simulink model "aircraft_control_model_v2"  (R2020b)
settings: Solver=ode1be  StartTime=0.0  StopTime=t  RelTol=1e-3
values from neighbouring files (symbols this model uses):
  A_ce_CG_14 = A_ce_CG_14(2:3,2:3)    [aircraft_control_model_initialisation_v2.m]
  A_ce_CG_24 = A_ce_CG_24(2:3,2:3)    [aircraft_control_model_initialisation_v2.m]
  A_ce_CG_34 = A_ce_CG_34(2:3,2:3)    [aircraft_control_model_initialisation_v2.m]
  A_sc_CG_10 = A_sc_CG_10(2:3,2:3)    [aircraft_control_model_initialisation_v2.m]
  A_sc_CG_22 = A_sc_CG_22(2:3,2:3)    [aircraft_control_model_initialisation_v2.m]
  A_sc_CG_29 = A_sc_CG_29(2:3,2:3)    [aircraft_control_model_initialisation_v2.m]
  A_sc_CG_36 = A_sc_CG_36(2:3,2:3)    [aircraft_control_model_initialisation_v2.m]
  A_sc_CG_55 = A_sc_CG_55(2:3,2:3)    [aircraft_control_model_initialisation_v2.m]
  actuator_rate = 115*pi/180    (= 2.00712863979)    [aircraft_control_model_initialisation_v2.m]
  ail_sat = 30*pi/180    (= 0.523598775598)    [aircraft_control_model_initialisation_v2.m]
  alpha0 = base_scout_aircraft_constants(16)    [aircraft_control_model_initialisation_v2.m]
  alpha0_ce = base_cessna_aircraft_constants(16)    [aircraft_control_model_initialisation_v2.m]
  alpha0tot_ce_CG_14 = consts_ce_CG_14(17)    [aircraft_control_model_initialisation_v2.m]
  alpha0tot_ce_CG_24 = consts_ce_CG_24(17)    [aircraft_control_model_initialisation_v2.m]
  alpha0tot_ce_CG_34 = consts_ce_CG_34(17)    [aircraft_control_model_initialisation_v2.m]
  alpha0tot_sc_CG_10 = consts_sc_CG_10(17)    [aircraft_control_model_initialisation_v2.m]
  alpha0tot_sc_CG_22 = consts_sc_CG_22(17)    [aircraft_control_model_initialisation_v2.m]
  alpha0tot_sc_CG_29 = consts_sc_CG_29(17)    [aircraft_control_model_initialisation_v2.m]
  alpha0tot_sc_CG_36 = consts_sc_CG_36(17)    [aircraft_control_model_initialisation_v2.m]
  alpha0tot_sc_CG_55 = consts_sc_CG_55(17)    [aircraft_control_model_initialisation_v2.m]
  alpha_ts = base_scout_aircraft_constants(19)    [aircraft_control_model_initialisation_v2.m]
  alpha_ts_ce = base_cessna_aircraft_constants(19)    [aircraft_control_model_initialisation_v2.m]
  alpha_ws = base_scout_aircraft_constants(18)    [aircraft_control_model_initialisation_v2.m]
  alpha_ws_ce = base_cessna_aircraft_constants(18)    [aircraft_control_model_initialisation_v2.m]
  AR_w = base_scout_aircraft_constants(8)    [aircraft_control_model_initialisation_v2.m]
  AR_w_ce = base_cessna_aircraft_constants(8)    [aircraft_control_model_initialisation_v2.m]
  b1 = base_scout_aircraft_constants(23)    [aircraft_control_model_initialisation_v2.m]
  b1_ce = base_cessna_aircraft_constants(23)    [aircraft_control_model_initialisation_v2.m]
  b2 = base_scout_aircraft_constants(24)    [aircraft_control_model_initialisation_v2.m]
  b2_ce = base_cessna_aircraft_constants(24)    [aircraft_control_model_initialisation_v2.m]
  b3 = base_scout_aircraft_constants(25)    [aircraft_control_model_initialisation_v2.m]
  b3_ce = base_cessna_aircraft_constants(25)    [aircraft_control_model_initialisation_v2.m]
  B_ce_CG_14 = B_ce_CG_14(2:3,1:1)    [aircraft_control_model_initialisation_v2.m]
  B_ce_CG_24 = B_ce_CG_24(2:3,1:1)    [aircraft_control_model_initialisation_v2.m]
  B_ce_CG_34 = B_ce_CG_34(2:3,1:1)    [aircraft_control_model_initialisation_v2.m]
  B_sc = B_sc(:,1)    [aircraft_control_model_initialisation_v2.m]
  B_sc_CG_10 = B_sc_CG_10(2:3,1:1)    [aircraft_control_model_initialisation_v2.m]
  B_sc_CG_22 = B_sc_CG_22(2:3,1:1)    [aircraft_control_model_initialisation_v2.m]
  B_sc_CG_29 = B_sc_CG_29(2:3,1:1)    [aircraft_control_model_initialisation_v2.m]
  B_sc_CG_36 = B_sc_CG_36(2:3,1:1)    [aircraft_control_model_initialisation_v2.m]
  B_sc_CG_55 = B_sc_CG_55(2:3,1:1)    [aircraft_control_model_initialisation_v2.m]
  beta_ce_CG_14 = consts_ce_CG_14(21)    [aircraft_control_model_initialisation_v2.m]
  beta_ce_CG_24 = consts_ce_CG_24(21)    [aircraft_control_model_initialisation_v2.m]
  beta_ce_CG_34 = consts_ce_CG_34(21)    [aircraft_control_model_initialisation_v2.m]
  beta_sc_CG_10 = consts_sc_CG_10(21)    [aircraft_control_model_initialisation_v2.m]
  beta_sc_CG_22 = consts_sc_CG_22(21)    [aircraft_control_model_initialisation_v2.m]
  beta_sc_CG_29 = consts_sc_CG_29(21)    [aircraft_control_model_initialisation_v2.m]
  beta_sc_CG_36 = consts_sc_CG_36(21)    [aircraft_control_model_initialisation_v2.m]
  beta_sc_CG_55 = consts_sc_CG_55(21)    [aircraft_control_model_initialisation_v2.m]
  c_e = base_scout_aircraft_constants(10)    [aircraft_control_model_initialisation_v2.m]
  c_e_ce = base_cessna_aircraft_constants(10)    [aircraft_control_model_initialisation_v2.m]
  Cm0 = base_scout_aircraft_constants(11)    [aircraft_control_model_initialisation_v2.m]
  control_surface_feedback = 10    [aircraft_control_model_initialisation_v2.m]
  dCL_w_dalpha = base_scout_aircraft_constants(14)    [aircraft_control_model_initialisation_v2.m]
  dCL_w_dalpha_ce = base_cessna_aircraft_constants(14)    [aircraft_control_model_initialisation_v2.m]
  dCLtot_dalpha = base_scout_aircraft_constants(15)    [aircraft_control_model_initialisation_v2.m]
  dCLtot_dalpha_ce = base_cessna_aircraft_constants(15)    [aircraft_control_model_initialisation_v2.m]
  dt = 1/100    (= 0.01)    [aircraft_control_model_initialisation_v2.m]
  elev_amplitude = 15*pi/180    (= 0.261799387799)    [aircraft_control_model_initialisation_v2.m]
  elev_cutoff = 35*pi/180    (= 0.610865238198)    [aircraft_control_model_initialisation_v2.m]
  elev_period = 1    [aircraft_control_model_initialisation_v2.m]
  elev_period_start = 5    [aircraft_control_model_initialisation_v2.m]
  elev_sat = 28*pi/180    (= 0.488692190558)    [aircraft_control_model_initialisation_v2.m]
  eta_ce_CG_14 = consts_ce_CG_14(22)    [aircraft_control_model_initialisation_v2.m]
  eta_ce_CG_24 = consts_ce_CG_24(22)    [aircraft_control_model_initialisation_v2.m]
  eta_ce_CG_34 = consts_ce_CG_34(22)    [aircraft_control_model_initialisation_v2.m]
  eta_sc_CG_10 = consts_sc_CG_10(22)    [aircraft_control_model_initialisation_v2.m]
  eta_sc_CG_22 = consts_sc_CG_22(22)    [aircraft_control_model_initialisation_v2.m]
  eta_sc_CG_29 = consts_sc_CG_29(22)    [aircraft_control_model_initialisation_v2.m]
  eta_sc_CG_36 = consts_sc_CG_36(22)    [aircraft_control_model_initialisation_v2.m]
  eta_sc_CG_55 = consts_sc_CG_55(22)    [aircraft_control_model_initialisation_v2.m]
  g = base_scout_aircraft_constants(3)    [aircraft_control_model_initialisation_v2.m]
  G = base_scout_aircraft_constants(26)    [aircraft_control_model_initialisation_v2.m]
  g_ce = base_cessna_aircraft_constants(3)    [aircraft_control_model_initialisation_v2.m]
  G_ce = base_cessna_aircraft_constants(26)    [aircraft_control_model_initialisation_v2.m]
  h0 = base_scout_aircraft_constants(13)    [aircraft_control_model_initialisation_v2.m]
  h_cg = base_scout_aircraft_constants(12)    [aircraft_control_model_initialisation_v2.m]
  K = base_scout_aircraft_constants(7)    [aircraft_control_model_initialisation_v2.m]
  l_m = base_scout_aircraft_constants(27)    [aircraft_control_model_initialisation_v2.m]
  l_m_ce = base_cessna_aircraft_constants(27)    [aircraft_control_model_initialisation_v2.m]
  m = base_scout_aircraft_constants(2)    [aircraft_control_model_initialisation_v2.m]
  m_ce = base_cessna_aircraft_constants(2)    [aircraft_control_model_initialisation_v2.m]
  modM = base_scout_aircraft_constants(30)    [aircraft_control_model_initialisation_v2.m]
  modM_ce = base_cessna_aircraft_constants(30)    [aircraft_control_model_initialisation_v2.m]
  n = base_scout_aircraft_constants(1)    [aircraft_control_model_initialisation_v2.m]    (also in xplane_data_decoder.m = data_input(6,2))
  ppgain_actuator_D = 1.076123507883140e+02    (= 107.612350788)    [aircraft_control_model_initialisation_v2.m]
  ppgain_actuator_P = 20.729870007825970    (= 20.7298700078)    [aircraft_control_model_initialisation_v2.m]
  ppgain_D = 0.637114873357555    (= 0.637114873358)    [aircraft_control_model_initialisation_v2.m]
  ppgain_P = -86.717674561182620    (= -86.7176745612)    [aircraft_control_model_initialisation_v2.m]
  r = base_scout_aircraft_constants(29)    [aircraft_control_model_initialisation_v2.m]
  r_ce = base_cessna_aircraft_constants(29)    [aircraft_control_model_initialisation_v2.m]
  rho = base_scout_aircraft_constants(4)    [aircraft_control_model_initialisation_v2.m]
  rho_ce = base_cessna_aircraft_constants(4)    [aircraft_control_model_initialisation_v2.m]
  rud_sat = 28*pi/180    (= 0.488692190558)    [aircraft_control_model_initialisation_v2.m]
  s_e = base_scout_aircraft_constants(9)    [aircraft_control_model_initialisation_v2.m]
  s_e_ce = base_cessna_aircraft_constants(9)    [aircraft_control_model_initialisation_v2.m]
  s_tp = base_scout_aircraft_constants(6)    [aircraft_control_model_initialisation_v2.m]
  s_w = base_scout_aircraft_constants(5)    [aircraft_control_model_initialisation_v2.m]
  s_w_ce = base_cessna_aircraft_constants(5)    [aircraft_control_model_initialisation_v2.m]
  tr = base_scout_aircraft_constants(28)    [aircraft_control_model_initialisation_v2.m]
  tr_ce = base_cessna_aircraft_constants(28)    [aircraft_control_model_initialisation_v2.m]
undefined symbols (not defined in the file or in its folder): A_sc
libraries: simulink x6, pid_lib x4, etargetslib x2, dspnetwork x2, aerolibanimutils x1, sldrtlib x1, cstblocks x1
(part 3 of 3)

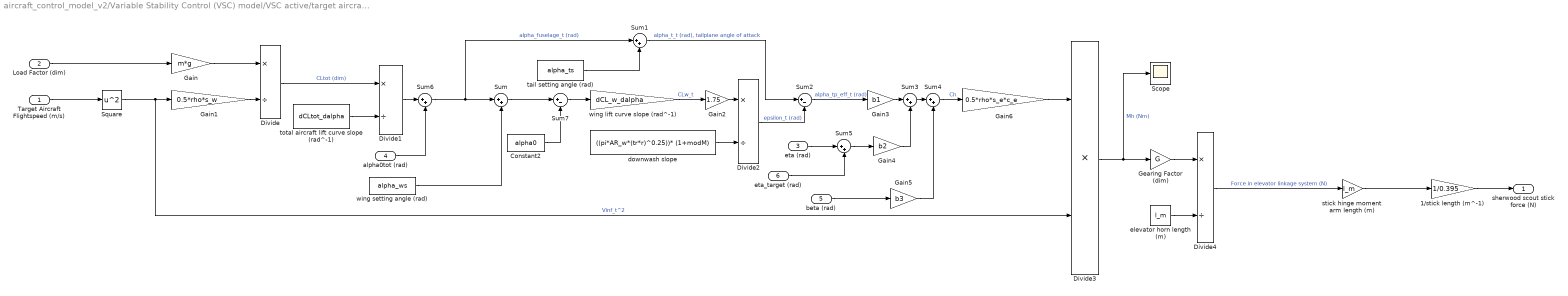
== system aircraft_control_model_v2/Variable Stability Control (VSC) model/VSC active/target aircraft state space selection/Target Aircraft Stick Force Calculation/sherwood scout stick force model/Subsystem ==
  Target Aircraft Flightspeed (m/s) : Inport
  Load Factor (dim) : Inport  Port=2
  eta (rad) : Inport  Port=3
  alpha0tot (rad) : Inport  Port=4
  beta (rad) : Inport  Port=5
  eta_target (rad) : Inport  Port=6
  1/stick length (m^-1) : Gain  Gain=1/0.395
  Constant2 : Constant  Value=alpha0
  Divide{,1..2,4} (4 alike) : Product  Inputs=*/
  Divide3 : Product  Inputs=**
  Gain : Gain  Gain=m*g
  Gain1 : Gain  Gain=0.5*rho*s_w
  Gain2 : Gain  Gain=1.75
  Gain3 : Gain  Gain=b1
  Gain4 : Gain  Gain=b2
  Gain5 : Gain  Gain=b3
  Gain6 : Gain  Gain=0.5*rho*s_e*c_e
  Gearing Factor (dim) : Gain  Gain=G
  Scope : Scope
  Square : Math  Operator=square  SaturateOnIntegerOverflow=on
  Sum{,1,3..6} (6 alike) : Sum  Inputs=|++
  Sum2 : Sum  Inputs=|+-
  Sum7 : Sum  Inputs=|+-
  downwash slope : Constant  Value=((pi*AR_w*(tr*r)^0.25))* (1+modM)
  elevator horn length (m) : Constant  Value=l_m
  stick hinge moment arm length (m) : Gain  Gain=l_m
  tail setting angle (rad) : Constant  Value=alpha_ts
  total aircraft lift curve slope (rad^-1) : Constant  Value=dCLtot_dalpha
  wing lift curve slope (rad^-1) : Gain  Gain=dCL_w_dalpha
  wing setting angle (rad) : Constant  Value=alpha_ws
  sherwood scout stick force (N) : Outport
  wires:
  stick hinge moment arm length (m)/1 -> 1/stick length (m^-1)/1
  Sum/1 -> Sum7/1
  Square/1 -> Gain1/1, Divide3/2  "Vinf_t^2"
  Constant2/1 -> Sum7/2
  Gain2/1 -> Divide2/1
  Gain1/1 -> Divide/2
  total aircraft lift curve slope (rad^-1)/1 -> Divide1/2
  tail setting angle (rad)/1 -> Sum1/2
  Gain4/1 -> Sum3/2
  1/stick length (m^-1)/1 -> sherwood scout stick force (N)/1
  Sum2/1 -> Gain3/1  "alpha_tp_eff_t (rad)"
  Gain/1 -> Divide/1
  Sum3/1 -> Sum4/1
  Divide3/1 -> Scope/1, Gearing Factor (dim)/1  "Mh (Nm)"
  Load Factor (dim)/1 -> Gain/1
  beta (rad)/1 -> Gain5/1
  Gain6/1 -> Divide3/1
  wing setting angle (rad)/1 -> Sum/2
  Sum1/1 -> Sum2/1  "alpha_t_t (rad), tailplane angle of attack"
  Gain3/1 -> Sum3/1
  Sum7/1 -> wing lift curve slope (rad^-1)/1
  Divide2/1 -> Sum2/2  "epsilon_t (rad)"
  wing lift curve slope (rad^-1)/1 -> Gain2/1  "CLw_t"
  Divide/1 -> Divide1/1  "CLtot (dim)"
  Gain5/1 -> Sum4/2
  Target Aircraft Flightspeed (m/s)/1 -> Square/1
  alpha0tot (rad)/1 -> Sum6/2
  Divide1/1 -> Sum6/1
  Sum6/1 -> Sum1/1, Sum/1  "alpha_fuselage_t (rad)"
  Gearing Factor (dim)/1 -> Divide4/1
  elevator horn length (m)/1 -> Divide4/2
  downwash slope/1 -> Divide2/2
  Sum4/1 -> Gain6/1  "Ch"
  Divide4/1 -> stick hinge moment arm length (m)/1  "Force in elevator linkage system (N)"
  eta (rad)/1 -> Sum5/1
  Sum5/1 -> Gain4/1
  eta_target (rad)/1 -> Sum5/2

== system aircraft_control_model_v2/Variable Stability Control (VSC) model/VSC active/target aircraft state space selection/Target Aircraft Stick Force Calculation/b-747-100 stick force model/Subsystem1/If Action Subsystem ==
  In1 : Inport
  Action Port : ActionPort  ActionPortLabel=else
  Feel System Gain for -5<=u1<=5 : Gain  Gain=43.9267
  Out1 : Outport
  wires:
  In1/1 -> Feel System Gain for -5<=u1<=5/1
  Feel System Gain for -5<=u1<=5/1 -> Out1/1

== system aircraft_control_model_v2/Variable Stability Control (VSC) model/VSC active/target aircraft state space selection/Target Aircraft Stick Force Calculation/b-747-100 stick force model/Subsystem1/If Action Subsystem1 ==
  In1 : Inport
  Action Port : ActionPort  ActionPortLabel=if(u1 > 2.5)
  Constant : Constant  Value=86.6986
  Feel System Gain for -5<=u1<=5 : Gain  Gain=9.5527
  Sum : Sum  Inputs=|++
  Out1 : Outport
  wires:
  In1/1 -> Feel System Gain for -5<=u1<=5/1
  Feel System Gain for -5<=u1<=5/1 -> Sum/1
  Constant/1 -> Sum/2
  Sum/1 -> Out1/1

== system aircraft_control_model_v2/Variable Stability Control (VSC) model/VSC active/target aircraft state space selection/Target Aircraft Stick Force Calculation/b-747-100 stick force model/Subsystem1/If Action Subsystem2 ==
  In1 : Inport
  Action Port : ActionPort  ActionPortLabel=elseif(u1 < -2.5)
  Constant : Constant  Value=-86.6986
  Feel System Gain for -5<=u1<=5 : Gain  Gain=9.5527
  Sum : Sum  Inputs=|++
  Out1 : Outport
  wires:
  In1/1 -> Feel System Gain for -5<=u1<=5/1
  Feel System Gain for -5<=u1<=5/1 -> Sum/1
  Constant/1 -> Sum/2
  Sum/1 -> Out1/1

== matlab function aircraft_control_model_v2/Receive Data from X-Plane (via UDP)/Subsystem1/MATLAB Function ==
  data: eta output; delta_a output; delta_r output; throttle output; delta_tt output; q output; roll_angle output; yaw_rate output; n output; vInd_kias output; data_input input
function[eta,delta_a,delta_r,throttle,delta_tt,q,roll_angle,yaw_rate,n,vInd_kias]=call_xplane_decoder(data_input)

[vInd_kias,~,n,q,roll_angle,yaw_rate,eta,delta_a,delta_r,throttle,delta_tt]=xplane_data_decoder(data_input);

== matlab function aircraft_control_model_v2/Send Control Commands to X-Plane (via UDP)/MATLAB Function ==
  data: elevator input; header output; control_surfaces_cmd output; throttle_cmd output; trim_cmd output; aileron input; rudder input; throttle input; trimtab input
function[header,control_surfaces_cmd,throttle_cmd,trim_cmd]=call_control_inputs_to_bytes(elevator,aileron,rudder,throttle,trimtab)

[header,control_surfaces_cmd,throttle_cmd,trim_cmd]=convert_control_inputs_to_bytes(elevator,aileron,rudder,throttle,trimtab);

end

== matlab function aircraft_control_model_v2/Control Inputs/predefined control input/Elevator Doublet Input/MATLAB Function ==
  data: u_in input; u_out output; clock_time input; elev_period input; elev_period_start input
function u_out =call_elevator_input(u_in,clock_time,elev_period,elev_period_start)
[u_out]=elevator_input(u_in,clock_time,elev_period,elev_period_start);
end

== matlab function aircraft_control_model_v2/Variable Stability Control (VSC) model/VSC active/system safety cutoffs/flight speed cutoff/MATLAB Function ==
  data: n input; Va output
function Va =call_flighspeedcutoff(n)

Va=flightspeedcutoff(n);
